simulink subsystem "April_Tag_Errors"  (R2023b)
settings: Solver=VariableStepAuto  StartTime=0.0  StopTime=10.0  RelTol=1e-3
undefined symbols (not defined in the file): AT_Target_Tag_11_Field_Angle, AT_Target_Tag_11_X, AT_Target_Tag_11_Y, AT_Target_Tag_12_Field_Angle, AT_Target_Tag_12_X, AT_Target_Tag_12_Y, AT_Target_Tag_13_Field_Angle, AT_Target_Tag_13_X, AT_Target_Tag_13_Y, AT_Target_Tag_14_Field_Angle, AT_Target_Tag_14_X, AT_Target_Tag_14_Y, AT_Target_Tag_15_Field_Angle, AT_Target_Tag_15_X, AT_Target_Tag_15_Y, AT_Target_Tag_16_Field_Angle, AT_Target_Tag_16_X, AT_Target_Tag_16_Y, AT_Target_Tag_5_Field_Angle, AT_Target_Tag_5_X, AT_Target_Tag_5_Y, AT_Target_Tag_6_Field_Angle, AT_Target_Tag_6_X, AT_Target_Tag_6_Y
settings Model: Creator=ander  LastModifiedBy=ander

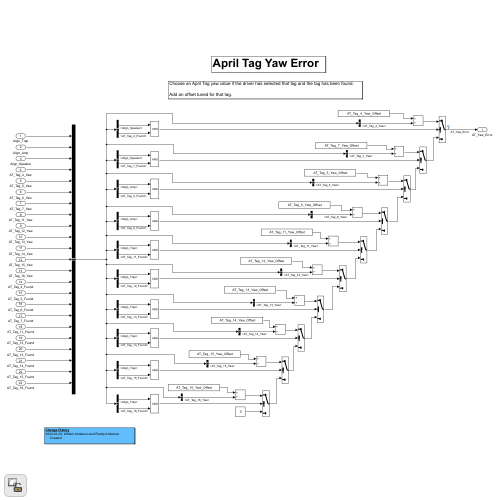
[thumbnail: Simulink's stored preview of the top-level diagram]
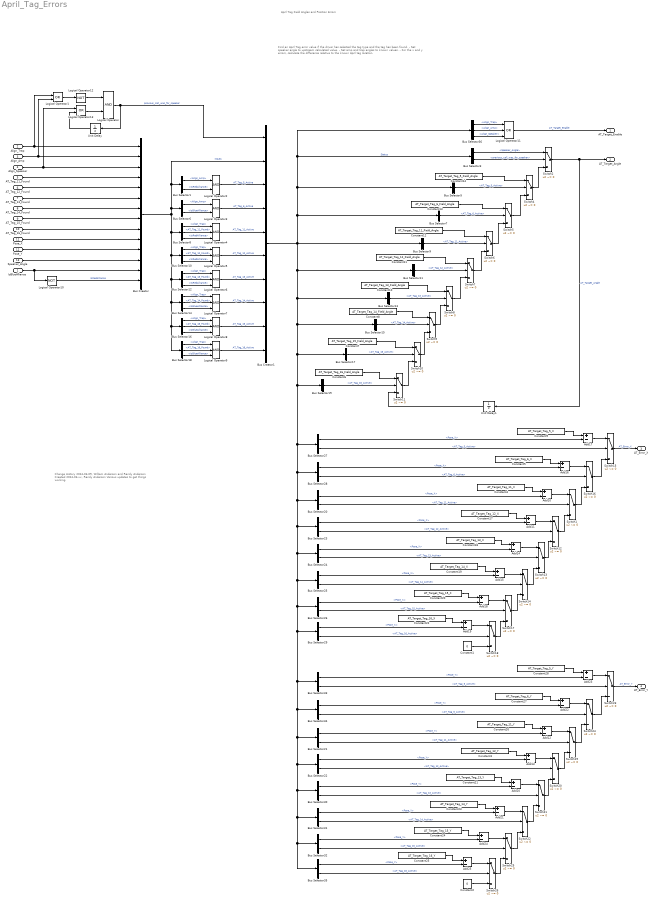
== system April_Tag_Errors ==
  note: April Tag
      | Field Angles and Position Errors
  note: Change History
      | 2024-03-09, William Anderson and Randy Anderson
      | Created
      | 2024-03-xx, Randy Anderson
      | Various updates to get things working.
  note: Find an April Tag error value if the driver has selected the tag type and the tag has been found.
      | - Set speaker angle to upstream calculated value.
      | - Set amp and trap angles to known values.
      | - For the x and y errors, calculate the difference relative to the known April tag location.
  IsBlueAlliance : Inport
  Align_Trap : Inport  Port=2
  Align_Amp : Inport  Port=3
  Align_Speaker : Inport  Port=4
  AT_Tag_11_Found : Inport  Port=5
  AT_Tag_12_Found : Inport  Port=6
  AT_Tag_13_Found : Inport  Port=7
  AT_Tag_14_Found : Inport  Port=8
  AT_Tag_15_Found : Inport  Port=9
  AT_Tag_16_Found : Inport  Port=10
  Pose_X : Inport  Port=11
  Pose_Y : Inport  Port=12
  Speaker_Angle : Inport  Port=13
  Add{10..25} (16 alike) : Sum  Inputs=+-
  Bus Creator : BusCreator  Inputs=14
  Bus Creator1 : BusCreator  Inputs=10
  Bus Selector1 : BusSelector  OutputSignals=Align_Amp,IsRedAlliance
  Bus Selector10 : BusSelector  OutputSignals=Align_Trap,AT_Tag_12_Found,IsRedAlliance
  Bus Selector11 : BusSelector  OutputSignals=AT_Tag_12_Active
  Bus Selector12 : BusSelector  OutputSignals=Align_Trap,AT_Tag_13_Found,IsRedAlliance
  Bus Selector13 : BusSelector  OutputSignals=AT_Tag_13_Active
  Bus Selector14 : BusSelector  OutputSignals=Align_Trap,AT_Tag_14_Found,IsBlueAlliance
  Bus Selector15 : BusSelector  OutputSignals=AT_Tag_14_Active
  Bus Selector16 : BusSelector  OutputSignals=Align_Trap,AT_Tag_15_Found,IsBlueAlliance
  Bus Selector17 : BusSelector  OutputSignals=AT_Tag_15_Active
  Bus Selector18 : BusSelector  OutputSignals=Align_Trap,AT_Tag_16_Found,IsBlueAlliance
  Bus Selector19 : BusSelector  OutputSignals=AT_Tag_16_Active
  Bus Selector20 : BusSelector  OutputSignals=Inputs.Pose_X,AT_Tag_11_Active
  Bus Selector21 : BusSelector  OutputSignals=Inputs.Pose_Y,AT_Tag_11_Active
  Bus Selector22 : BusSelector  OutputSignals=Inputs.Pose_Y,AT_Tag_12_Active
  Bus Selector23 : BusSelector  OutputSignals=Inputs.Pose_X,AT_Tag_12_Active
  Bus Selector24 : BusSelector  OutputSignals=Inputs.Pose_X,AT_Tag_13_Active
  Bus Selector25 : BusSelector  OutputSignals=Inputs.Pose_X,AT_Tag_14_Active
  Bus Selector26 : BusSelector  OutputSignals=Inputs.Pose_X,AT_Tag_15_Active
  Bus Selector27 : BusSelector  OutputSignals=Inputs.Pose_X,AT_Tag_5_Active
  Bus Selector28 : BusSelector  OutputSignals=Inputs.Pose_X,AT_Tag_6_Active
  Bus Selector29 : BusSelector  OutputSignals=Inputs.Pose_X,AT_Tag_16_Active
  Bus Selector3 : BusSelector  OutputSignals=Inputs.Speaker_Angle,previous_call_was_for_speaker
  Bus Selector30 : BusSelector  OutputSignals=Inputs.Pose_Y,AT_Tag_13_Active
  Bus Selector31 : BusSelector  OutputSignals=Inputs.Pose_Y,AT_Tag_14_Active
  Bus Selector32 : BusSelector  OutputSignals=Inputs.Pose_Y,AT_Tag_15_Active
  Bus Selector33 : BusSelector  OutputSignals=Inputs.Pose_Y,AT_Tag_5_Active
  Bus Selector34 : BusSelector  OutputSignals=Inputs.Pose_Y,AT_Tag_6_Active
  Bus Selector35 : BusSelector  OutputSignals=Inputs.Pose_Y,AT_Tag_16_Active
  Bus Selector36 : BusSelector  OutputSignals=Inputs.Align_Trap,Inputs.Align_Amp,Inputs.Align_Speaker
  Bus Selector5 : BusSelector  OutputSignals=AT_Tag_5_Active
  Bus Selector6 : BusSelector  OutputSignals=Align_Amp,IsBlueAlliance
  Bus Selector7 : BusSelector  OutputSignals=AT_Tag_6_Active
  Bus Selector8 : BusSelector  OutputSignals=Align_Trap,AT_Tag_11_Found,IsRedAlliance
  Bus Selector9 : BusSelector  OutputSignals=AT_Tag_11_Active
  Constant1 : Constant  Value=0
  Constant10 : Constant  Value=AT_Target_Tag_13_Field_Angle
  Constant11 : Constant  Value=AT_Target_Tag_12_Field_Angle
  Constant12 : Constant  Value=AT_Target_Tag_11_Field_Angle
  Constant13 : Constant  Value=AT_Target_Tag_6_Field_Angle
  Constant14 : Constant  Value=AT_Target_Tag_5_Field_Angle
  Constant17 : Constant  Value=AT_Target_Tag_12_X
  Constant18 : Constant  Value=AT_Target_Tag_13_X
  Constant19 : Constant  Value=AT_Target_Tag_14_X
  Constant2 : Constant  Value=0
  Constant20 : Constant  Value=AT_Target_Tag_15_X
  Constant21 : Constant  Value=AT_Target_Tag_13_Y
  Constant22 : Constant  Value=AT_Target_Tag_16_X
  Constant23 : Constant  Value=AT_Target_Tag_14_Y
  Constant24 : Constant  Value=AT_Target_Tag_15_Y
  Constant25 : Constant  Value=AT_Target_Tag_16_Y
  Constant26 : Constant  Value=AT_Target_Tag_11_Y
  Constant27 : Constant  Value=AT_Target_Tag_6_Y
  Constant28 : Constant  Value=AT_Target_Tag_5_Y
  Constant3 : Constant  Value=AT_Target_Tag_12_Y
  Constant4 : Constant  Value=AT_Target_Tag_11_X
  Constant5 : Constant  Value=AT_Target_Tag_6_X
  Constant6 : Constant  Value=AT_Target_Tag_16_Field_Angle
  Constant7 : Constant  Value=AT_Target_Tag_15_Field_Angle
  Constant8 : Constant  Value=AT_Target_Tag_14_Field_Angle
  Constant9 : Constant  Value=AT_Target_Tag_5_X
  Logical Operator : Logic  AllPortsSameDT=off  OutDataTypeStr=boolean
  Logical Operator1 : Logic  Operator=OR  AllPortsSameDT=off  OutDataTypeStr=boolean
  Logical Operator10 : Logic  Operator=NOT  AllPortsSameDT=off  OutDataTypeStr=boolean
  Logical Operator11 : Logic  Operator=OR  Inputs=3  AllPortsSameDT=off  OutDataTypeStr=boolean
  Logical Operator12 : Logic  Operator=NOT  AllPortsSameDT=off  OutDataTypeStr=boolean
  Logical Operator13 : Logic  Operator=OR  AllPortsSameDT=off  OutDataTypeStr=boolean
  Logical Operator2 : Logic  AllPortsSameDT=off  OutDataTypeStr=boolean
  Logical Operator3 : Logic  AllPortsSameDT=off  OutDataTypeStr=boolean
  Logical Operator{4..9} (6 alike) : Logic  Inputs=3  AllPortsSameDT=off  OutDataTypeStr=boolean
  Switch{1..2,4..26} (25 alike) : Switch  Criteria=u2 ~= 0  SaturateOnIntegerOverflow=off  InputSameDT=off
  Unit Delay : UnitDelay  SampleTime=-1  HasFrameUpgradeWarning=on
  Unit Delay1 : UnitDelay  SampleTime=-1  HasFrameUpgradeWarning=on
  AT_Target_Enable : Outport
  AT_Target_Angle : Outport  Port=2
  AT_Error_X : Outport  Port=3
  AT_Error_Y : Outport  Port=4
  wires:
  Switch23/1 -> AT_Error_Y/1  "AT_Error_Y"
  Bus Selector32/1 -> Add24/2  "<Pose_Y>"
  Constant27/1 -> Add22/1
  Constant28/1 -> Add23/1
  Bus Selector32/2 -> Switch25/2  "<AT_Tag_15_Active>"
  Add22/1 -> Switch24/1
  Bus Selector30/1 -> Add20/2  "<Pose_Y>"
  Add23/1 -> Switch23/1
  Bus Selector22/1 -> Add13/2  "<Pose_Y>"
  Switch24/1 -> Switch23/3
  Constant21/1 -> Add20/1
  Bus Selector33/1 -> Add23/2  "<Pose_Y>"
  Bus Selector34/1 -> Add22/2  "<Pose_Y>"
  Switch22/1 -> Switch21/3
  Bus Selector35/1 -> Add25/2  "<Pose_Y>"
  Bus Selector22/2 -> Switch20/2  "<AT_Tag_12_Active>"
  Bus Selector33/2 -> Switch23/2  "<AT_Tag_5_Active>"
  Bus Selector34/2 -> Switch24/2  "<AT_Tag_6_Active>"
  Add21/1 -> Switch22/1
  Switch21/1 -> Switch20/3
  Switch25/1 -> Switch22/3
  Add25/1 -> Switch26/1
  Switch26/1 -> Switch25/3
  Constant2/1 -> Switch26/3
  Add13/1 -> Switch20/1
  Constant3/1 -> Add13/1
  Bus Selector31/2 -> Switch22/2  "<AT_Tag_14_Active>"
  Bus Selector35/2 -> Switch26/2  "<AT_Tag_16_Active>"
  Constant25/1 -> Add25/1
  Add24/1 -> Switch25/1
  Switch20/1 -> Switch19/3
  Constant24/1 -> Add24/1
  Constant23/1 -> Add21/1
  Bus Selector21/1 -> Add12/2  "<Pose_Y>"
  Bus Selector30/2 -> Switch21/2  "<AT_Tag_13_Active>"
  Add20/1 -> Switch21/1
  Bus Selector21/2 -> Switch19/2  "<AT_Tag_11_Active>"
  Switch19/1 -> Switch24/3
  Add12/1 -> Switch19/1
  Constant26/1 -> Add12/1
  Bus Selector31/1 -> Add21/2  "<Pose_Y>"
  Constant1/1 -> Switch18/3
  Switch18/1 -> Switch17/3
  Switch17/1 -> Switch14/3
  Switch14/1 -> Switch13/3
  Switch13/1 -> Switch12/3
  Switch12/1 -> Switch1/3
  Switch1/1 -> Switch16/3
  Constant20/1 -> Add18/1
  Constant22/1 -> Add19/1
  Add18/1 -> Switch17/1
  Bus Selector26/1 -> Add18/2  "<Pose_X>"
  Bus Selector26/2 -> Switch17/2  "<AT_Tag_15_Active>"
  Bus Selector29/2 -> Switch18/2  "<AT_Tag_16_Active>"
  Bus Selector29/1 -> Add19/2  "<Pose_X>"
  Add19/1 -> Switch18/1
  Add15/1 -> Switch14/1
  Bus Selector25/2 -> Switch14/2  "<AT_Tag_14_Active>"
  Bus Selector25/1 -> Add15/2  "<Pose_X>"
  Constant19/1 -> Add15/1
  Add14/1 -> Switch13/1
  Bus Selector24/2 -> Switch13/2  "<AT_Tag_13_Active>"
  Bus Selector24/1 -> Add14/2  "<Pose_X>"
  Constant18/1 -> Add14/1
  Constant17/1 -> Add11/1
  Add11/1 -> Switch12/1
  Bus Selector23/1 -> Add11/2  "<Pose_X>"
  Bus Selector23/2 -> Switch12/2  "<AT_Tag_12_Active>"
  Constant4/1 -> Add10/1
  Add10/1 -> Switch1/1
  Bus Selector20/1 -> Add10/2  "<Pose_X>"
  Bus Selector20/2 -> Switch1/2  "<AT_Tag_11_Active>"
  Bus Selector28/2 -> Switch16/2  "<AT_Tag_6_Active>"
  Bus Selector28/1 -> Add16/2  "<Pose_X>"
  Bus Selector27/2 -> Switch15/2  "<AT_Tag_5_Active>"
  Bus Selector27/1 -> Add17/2  "<Pose_X>"
  Switch8/1 -> Switch7/3
  Bus Selector18/1 -> Logical Operator9/1  "<Align_Trap>"
  Switch4/1 -> Switch2/3
  Bus Creator/1 -> Bus Selector8/1, Bus Selector12/1, Bus Selector14/1, Bus Selector16/1, Bus Selector18/1, Bus Selector10/1, Bus Selector6/1, Bus Selector1/1, Bus Creator1/2  "Inputs"
  Bus Selector16/1 -> Logical Operator8/1  "<Align_Trap>"
  Switch9/1 -> Switch8/3
  Switch11/1 -> Switch10/3
  Switch6/1 -> Switch5/3
  Bus Selector10/1 -> Logical Operator5/1  "<Align_Trap>"
  Bus Selector8/2 -> Logical Operator4/2  "<AT_Tag_11_Found>"
  Align_Speaker/1 -> Bus Creator/3, Logical Operator13/1
  Bus Selector12/1 -> Logical Operator6/1  "<Align_Trap>"
  Bus Selector16/2 -> Logical Operator8/2  "<AT_Tag_15_Found>"
  Bus Selector18/2 -> Logical Operator9/2  "<AT_Tag_16_Found>"
  Bus Selector6/1 -> Logical Operator3/1  "<Align_Amp>"
  Switch5/1 -> Switch4/3
  Bus Selector12/2 -> Logical Operator6/2  "<AT_Tag_13_Found>"
  Switch10/1 -> Switch9/3
  Bus Selector8/1 -> Logical Operator4/1  "<Align_Trap>"
  Switch7/1 -> Switch6/3
  Bus Selector10/2 -> Logical Operator5/2  "<AT_Tag_12_Found>"
  Bus Selector1/1 -> Logical Operator2/1  "<Align_Amp>"
  Bus Selector14/2 -> Logical Operator7/2  "<AT_Tag_14_Found>"
  Bus Selector14/1 -> Logical Operator7/1  "<Align_Trap>"
  Align_Trap/1 -> Bus Creator/1, Logical Operator1/1
  Align_Amp/1 -> Bus Creator/2, Logical Operator1/2
  Logical Operator2/1 -> Bus Creator1/3  "AT_Tag_5_Active"
  Logical Operator3/1 -> Bus Creator1/4  "AT_Tag_6_Active"
  Logical Operator4/1 -> Bus Creator1/5  "AT_Tag_11_Active"
  Logical Operator5/1 -> Bus Creator1/6  "AT_Tag_12_Active"
  Logical Operator6/1 -> Bus Creator1/7  "AT_Tag_13_Active"
  Logical Operator7/1 -> Bus Creator1/8  "AT_Tag_14_Active"
  Logical Operator8/1 -> Bus Creator1/9  "AT_Tag_15_Active"
  Logical Operator9/1 -> Bus Creator1/10  "AT_Tag_16_Active"
  Bus Selector5/1 -> Switch4/2  "<AT_Tag_5_Active>"
  Bus Selector7/1 -> Switch5/2  "<AT_Tag_6_Active>"
  Bus Selector9/1 -> Switch6/2  "<AT_Tag_11_Active>"
  Bus Selector11/1 -> Switch7/2  "<AT_Tag_12_Active>"
  Bus Selector13/1 -> Switch8/2  "<AT_Tag_13_Active>"
  Bus Selector15/1 -> Switch9/2  "<AT_Tag_14_Active>"
  Bus Selector17/1 -> Switch10/2  "<AT_Tag_15_Active>"
  Bus Selector19/1 -> Switch11/2  "<AT_Tag_16_Active>"
  Switch16/1 -> Switch15/3
  Constant9/1 -> Add17/1
  Add17/1 -> Switch15/1
  Bus Creator1/1 -> Bus Selector9/1, Bus Selector7/1, Bus Selector5/1, Bus Selector3/1, Bus Selector36/1, Bus Selector11/1, Bus Selector19/1, Bus Selector28/1, Bus Selector20/1, Bus Selector23/1, Bus Selector24/1, Bus Selector25/1, Bus Selector26/1, Bus Selector29/1, Bus Selector34/1, Bus Selector21/1, Bus Selector22/1, Bus Selector30/1, Bus Selector31/1, Bus Selector32/1, Bus Selector35/1, Bus Selector33/1, Bus Selector27/1, Bus Selector17/1, Bus Selector15/1, Bus Selector13/1  "Status"
  Add16/1 -> Switch16/1
  Constant5/1 -> Add16/1
  Switch15/1 -> AT_Error_X/1  "AT_Error_X"
  Switch2/1 -> AT_Target_Angle/1, Unit Delay1/1  "AT_Target_Angle"
  AT_Tag_11_Found/1 -> Bus Creator/4
  AT_Tag_12_Found/1 -> Bus Creator/5
  AT_Tag_13_Found/1 -> Bus Creator/6
  AT_Tag_14_Found/1 -> Bus Creator/7
  AT_Tag_15_Found/1 -> Bus Creator/8
  AT_Tag_16_Found/1 -> Bus Creator/9
  Pose_X/1 -> Bus Creator/10
  Pose_Y/1 -> Bus Creator/11
  Speaker_Angle/1 -> Bus Creator/12
  IsBlueAlliance/1 -> Bus Creator/13, Logical Operator10/1
  Logical Operator10/1 -> Bus Creator/14  "IsRedAlliance"
  Bus Selector1/2 -> Logical Operator2/2  "<IsRedAlliance>"
  Bus Selector6/2 -> Logical Operator3/2  "<IsBlueAlliance>"
  Bus Selector10/3 -> Logical Operator5/3  "<IsRedAlliance>"
  Bus Selector8/3 -> Logical Operator4/3  "<IsRedAlliance>"
  Bus Selector12/3 -> Logical Operator6/3  "<IsRedAlliance>"
  Bus Selector14/3 -> Logical Operator7/3  "<IsBlueAlliance>"
  Bus Selector16/3 -> Logical Operator8/3  "<IsBlueAlliance>"
  Bus Selector18/3 -> Logical Operator9/3  "<IsBlueAlliance>"
  Bus Selector3/1 -> Switch2/1  "<Speaker_Angle>"
  Constant14/1 -> Switch4/1
  Constant13/1 -> Switch5/1
  Constant12/1 -> Switch6/1
  Constant11/1 -> Switch7/1
  Constant10/1 -> Switch8/1
  Constant8/1 -> Switch9/1
  Constant7/1 -> Switch10/1
  Constant6/1 -> Switch11/1
  Bus Selector36/1 -> Logical Operator11/1  "<Align_Trap>"
  Bus Selector36/2 -> Logical Operator11/2  "<Align_Amp>"
  Bus Selector36/3 -> Logical Operator11/3  "<Align_Speaker>"
  Logical Operator11/1 -> AT_Target_Enable/1  "AT_Target_Enable"
  Logical Operator1/1 -> Logical Operator12/1
  Logical Operator12/1 -> Logical Operator/1
  Logical Operator13/1 -> Logical Operator/2
  Logical Operator/1 -> Unit Delay/1, Bus Creator1/1  "previous_call_was_for_speaker"
  Unit Delay/1 -> Logical Operator13/2
  Bus Selector3/2 -> Switch2/2  "<previous_call_was_for_speaker>"
  Unit Delay1/1 -> Switch11/3
